simulink model "BMS_Model"  (R2023b)
settings: Solver=ode45  StartTime=0.0  StopTime=1180  RelTol=1e-3
values from neighbouring files (symbols this model uses):
  C1_LUT = [1913.6,12447,30609 ... (first row only)    [Cell_Data_Script.m]
  Capacity_LUT = [28.01,27.63,27.64]    [Cell_Data_Script.m]
  cell_area = cell_length*cell_width    (= 0.02678)    [Cell_Data_Script.m]
  cell_cp_heat = 830    [Cell_Data_Script.m]
  cell_mass = 0.354    [Cell_Data_Script.m]
  Em_LUT = [3.49,3.51,3.52;3.55,3.56,3.56 ... (first row only)    [Cell_Data_Script.m]
  h_conv = 10    [Cell_Data_Script.m]
  R0_LUT = [0.0117,0.0085,0.0090;0.0110,0.0085,0.0090 ... (first row only)    [Cell_Data_Script.m]
  R1_LUT = [0.0109,0.0029,0.0013;0.0069,0.0024,0.0012 ... (first row only)    [Cell_Data_Script.m]
  SOC_LUT = [0;0.1;0.25;0.5;0.75;0.9;1.0]    [Cell_Data_Script.m]
  T_init = 293.15    [Cell_Data_Script.m]
  Temperature_LUT = [278.15,293.15,313.15]    [Cell_Data_Script.m]
settings Model: Creator=marri  LastModifiedBy=marri

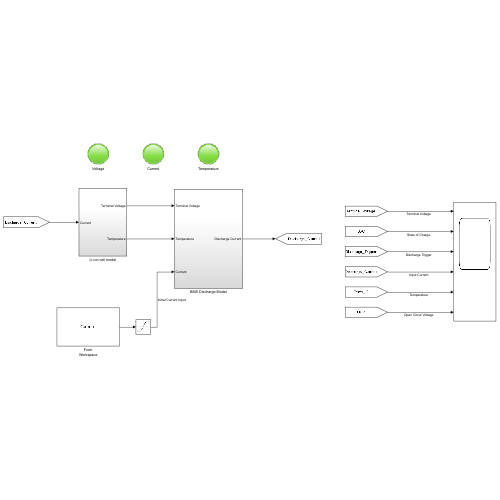
[thumbnail: Simulink's stored preview of the top-level diagram]
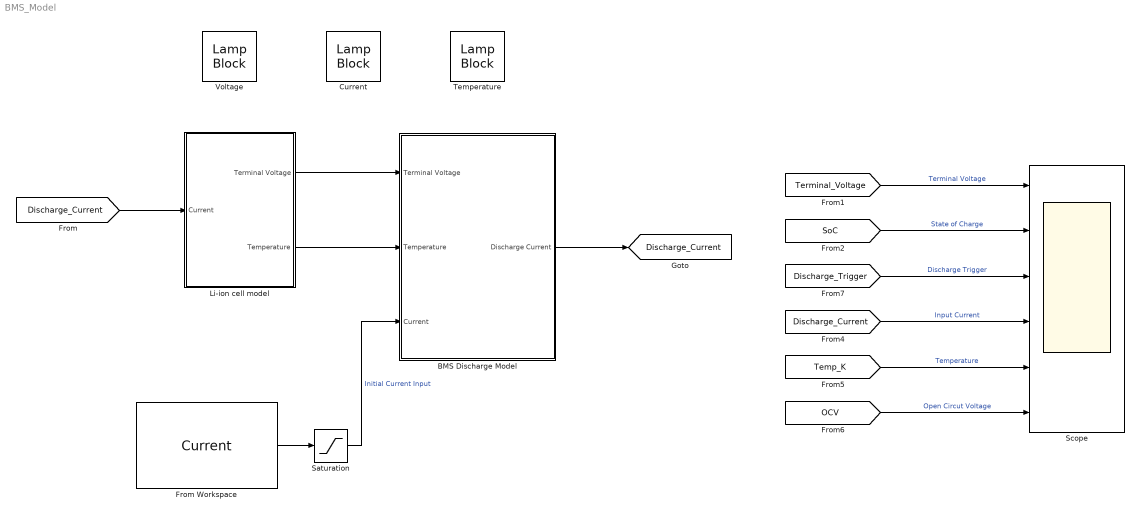
== system BMS_Model ==
  BMS Discharge Model : Subsystem
  Current : LampBlock  LabelPosition=Hide
  From Workspace : FromWorkspace  VariableName=Current
  Li-ion cell model : Subsystem
  Saturation : Saturate  UpperLimit=+inf  LowerLimit=0
  Scope : Scope  NumInputPorts=6
  Temperature : LampBlock  LabelPosition=Hide
  Voltage : LampBlock  LabelPosition=Hide
  tag scope: Discharge_Current=global
  wires:
  From Workspace/1 -> Saturation/1
  Saturation/1 -> BMS Discharge Model/3(Current)  "Initial Current Input"
  BMS Discharge Model/1(Discharge Current) -> [Discharge_Current]
  [Discharge_Current] -> Li-ion cell model/1(Current)
  Li-ion cell model/1(Terminal Voltage) -> BMS Discharge Model/1(Terminal Voltage)
  Li-ion cell model/2(Temperature) -> BMS Discharge Model/2(Temperature)
  [Terminal_Voltage] -> Scope/1  "Terminal Voltage"
  [SoC] -> Scope/2  "State of Charge"
  [Discharge_Current] -> Scope/4  "Input Current"
  [Temp_K] -> Scope/5  "Temperature"
  [OCV] -> Scope/6  "Open Circut Voltage"
  [Discharge_Trigger] -> Scope/3  "Discharge Trigger"

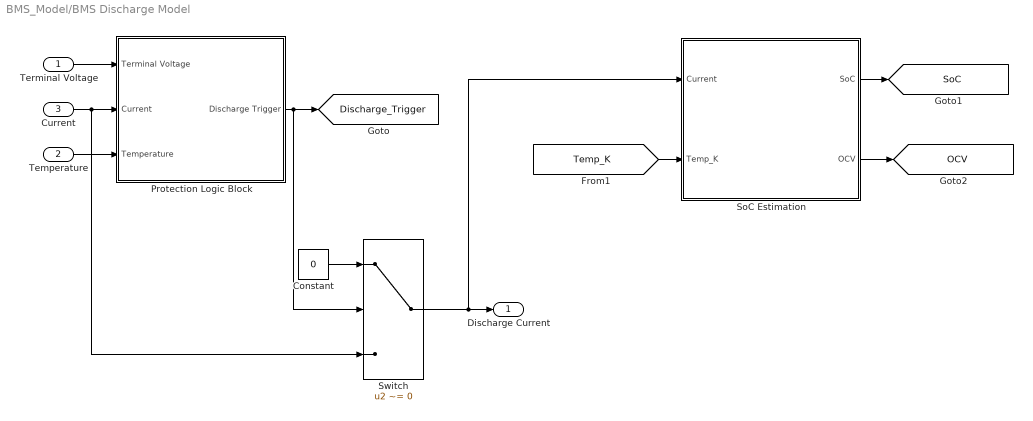
== system BMS_Model/BMS Discharge Model ==
  Terminal Voltage : Inport
  Temperature : Inport  Port=2
  Current : Inport  Port=3
  Constant : Constant  Value=0
  Protection Logic Block : Subsystem
  SoC Estimation : Subsystem
  Switch : Switch  Criteria=u2 ~= 0  SaturateOnIntegerOverflow=off  InputSameDT=off
  Discharge Current : Outport
  tag scope: Discharge_Trigger=global, OCV=global, SoC=global
  wires:
  Terminal Voltage/1 -> Protection Logic Block/1(Terminal Voltage)
  Current/1 -> Switch/3, Protection Logic Block/2(Current)
  Temperature/1 -> Protection Logic Block/3(Temperature)
  Protection Logic Block/1(Discharge Trigger) -> Switch/2, [Discharge_Trigger]
  Constant/1 -> Switch/1
  Switch/1 -> Discharge Current/1, SoC Estimation/1(Current)
  [Temp_K] -> SoC Estimation/2(Temp_K)
  SoC Estimation/1(SoC) -> [SoC]
  SoC Estimation/2(OCV) -> [OCV]

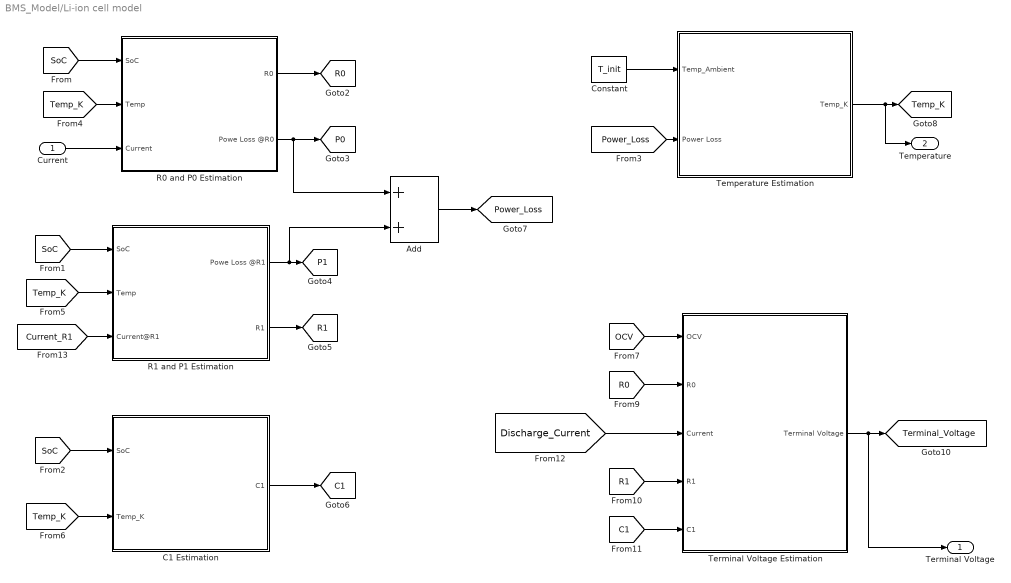
== system BMS_Model/Li-ion cell model ==
  Current : Inport
  Add : Sum
  C1 Estimation : Subsystem
  Constant : Constant  Value=T_init
  R0 and P0 Estimation : Subsystem
  R1 and P1 Estimation : Subsystem
  Temperature Estimation : Subsystem
  Terminal Voltage Estimation : Subsystem
  Terminal Voltage : Outport
  Temperature : Outport  Port=2
  tag scope: C1=global, P0=global, P1=global, Power_Loss=global, R0=global, R1=global, Temp_K=global, Terminal_Voltage=global
  wires:
  [SoC] -> R0 and P0 Estimation/1(SoC)
  [SoC] -> R1 and P1 Estimation/1(SoC)
  R0 and P0 Estimation/1(R0) -> [R0]
  R0 and P0 Estimation/2(Powe Loss @R0) -> Add/1, [P0]
  R1 and P1 Estimation/1(Powe Loss @R1) -> Add/2, [P1]
  R1 and P1 Estimation/2(R1) -> [R1]
  [SoC] -> C1 Estimation/1(SoC)
  C1 Estimation/1(C1) -> [C1]
  Add/1 -> [Power_Loss]
  Constant/1 -> Temperature Estimation/1(Temp_Ambient)
  [Power_Loss] -> Temperature Estimation/2(Power Loss)
  Temperature Estimation/1(Temp_K) -> Temperature/1, [Temp_K]
  [Temp_K] -> R0 and P0 Estimation/2(Temp)
  [Temp_K] -> R1 and P1 Estimation/2(Temp)
  [Temp_K] -> C1 Estimation/2(Temp_K)
  [R0] -> Terminal Voltage Estimation/2(R0)
  [R1] -> Terminal Voltage Estimation/4(R1)
  [C1] -> Terminal Voltage Estimation/5(C1)
  [Discharge_Current] -> Terminal Voltage Estimation/3(Current)
  [Current_R1] -> R1 and P1 Estimation/3(Current@R1)
  Terminal Voltage Estimation/1(Terminal Voltage) -> Terminal Voltage/1, [Terminal_Voltage]
  Current/1 -> R0 and P0 Estimation/3(Current)
  [OCV] -> Terminal Voltage Estimation/1(OCV)

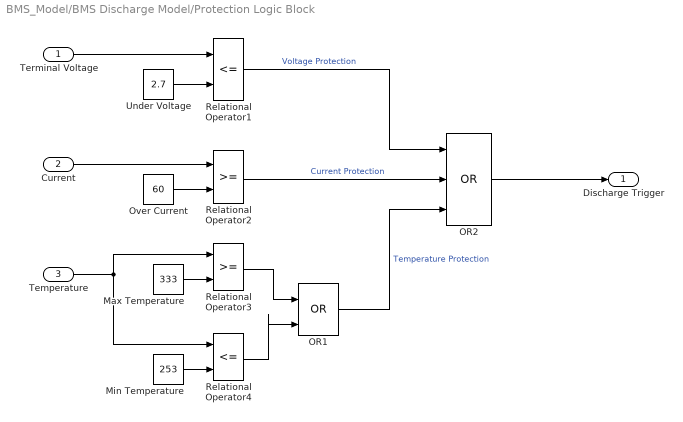
== system BMS_Model/BMS Discharge Model/Protection Logic Block ==
  Terminal Voltage : Inport
  Current : Inport  Port=2
  Temperature : Inport  Port=3
  Max Temperature : Constant  Value=333
  Min Temperature : Constant  Value=253
  OR1 : Logic  Operator=OR  IconShape=distinctive  AllPortsSameDT=off  OutDataTypeStr=boolean
  OR2 : Logic  Operator=OR  Inputs=3  IconShape=distinctive  AllPortsSameDT=off  OutDataTypeStr=boolean
  Over Current : Constant  Value=60
  Relational Operator1 : RelationalOperator  Operator=<=  OutDataTypeStr=boolean  RndMeth=Simplest  InputSameDT=off
  Relational Operator2 : RelationalOperator  OutDataTypeStr=boolean  RndMeth=Simplest  InputSameDT=off
  Relational Operator3 : RelationalOperator  OutDataTypeStr=boolean  RndMeth=Simplest  InputSameDT=off
  Relational Operator4 : RelationalOperator  Operator=<=  OutDataTypeStr=boolean  RndMeth=Simplest  InputSameDT=off
  Under Voltage : Constant  Value=2.7
  Discharge Trigger : Outport
  wires:
  Terminal Voltage/1 -> Relational Operator1/1
  Under Voltage/1 -> Relational Operator1/2
  Current/1 -> Relational Operator2/1
  Over Current/1 -> Relational Operator2/2
  Temperature/1 -> Relational Operator4/1, Relational Operator3/1
  Max Temperature/1 -> Relational Operator3/2
  Min Temperature/1 -> Relational Operator4/2
  Relational Operator3/1 -> OR1/1
  Relational Operator4/1 -> OR1/2
  Relational Operator2/1 -> OR2/2  "Current Protection"
  OR1/1 -> OR2/3  "Temperature Protection"
  OR2/1 -> Discharge Trigger/1
  Relational Operator1/1 -> OR2/1  "Voltage Protection"

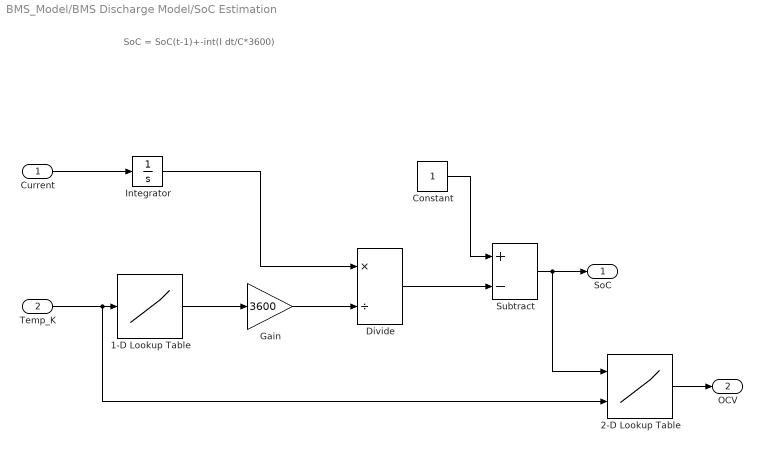
== system BMS_Model/BMS Discharge Model/SoC Estimation ==
  note: SoC = SoC(t-1)+-int(I dt/C*3600)
  Current : Inport
  Temp_K : Inport  Port=2
  1-D Lookup Table : Lookup_n-D  NumberOfTableDimensions=1  BreakpointsForDimension1=Temperature_LUT  Table=Capacity_LUT  InternalRulePriority=Speed  RndMeth=Simplest
  2-D Lookup Table : Lookup_n-D  BreakpointsForDimension1=SOC_LUT  BreakpointsForDimension2=Temperature_LUT  Table=Em_LUT  InternalRulePriority=Speed  RndMeth=Simplest
      settings: InputPortMap=u0,u1
  Constant : Constant
  Divide : Product  Inputs=*/
  Gain : Gain  Gain=3600
  Integrator : Integrator
  Subtract : Sum  Inputs=+-
  SoC : Outport
  OCV : Outport  Port=2
  wires:
  Temp_K/1 -> 2-D Lookup Table/2, 1-D Lookup Table/1
  1-D Lookup Table/1 -> Gain/1
  Current/1 -> Integrator/1
  Gain/1 -> Divide/2
  Integrator/1 -> Divide/1
  Divide/1 -> Subtract/2
  Constant/1 -> Subtract/1
  Subtract/1 -> 2-D Lookup Table/1, SoC/1
  2-D Lookup Table/1 -> OCV/1

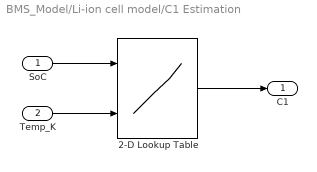
== system BMS_Model/Li-ion cell model/C1 Estimation ==
  SoC : Inport
  Temp_K : Inport  Port=2
  2-D Lookup Table : Lookup_n-D  BreakpointsForDimension1=SOC_LUT  BreakpointsForDimension2=Temperature_LUT  Table=C1_LUT  InternalRulePriority=Speed  RndMeth=Simplest
      settings: InputPortMap=u0,u1
  C1 : Outport
  wires:
  SoC/1 -> 2-D Lookup Table/1
  Temp_K/1 -> 2-D Lookup Table/2
  2-D Lookup Table/1 -> C1/1

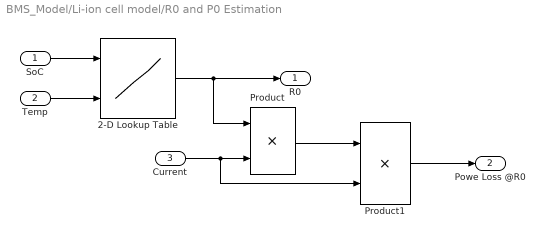
== system BMS_Model/Li-ion cell model/R0 and P0 Estimation ==
  SoC : Inport
  Temp : Inport  Port=2
  Current : Inport  Port=3
  2-D Lookup Table : Lookup_n-D  BreakpointsForDimension1=SOC_LUT  BreakpointsForDimension2=Temperature_LUT  Table=R0_LUT  InternalRulePriority=Speed  RndMeth=Simplest
      settings: InputPortMap=u0,u1
  Product : Product
  Product1 : Product
  R0 : Outport
  Powe Loss @R0 : Outport  Port=2
  wires:
  SoC/1 -> 2-D Lookup Table/1
  Temp/1 -> 2-D Lookup Table/2
  2-D Lookup Table/1 -> R0/1, Product/1
  Current/1 -> Product/2, Product1/2
  Product/1 -> Product1/1
  Product1/1 -> Powe Loss @R0/1

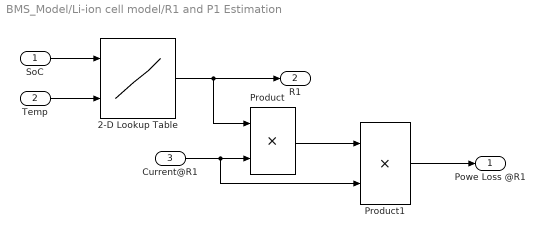
== system BMS_Model/Li-ion cell model/R1 and P1 Estimation ==
  SoC : Inport
  Temp : Inport  Port=2
  Current@R1 : Inport  Port=3
  2-D Lookup Table : Lookup_n-D  BreakpointsForDimension1=SOC_LUT  BreakpointsForDimension2=Temperature_LUT  Table=R1_LUT  InternalRulePriority=Speed  RndMeth=Simplest
      settings: InputPortMap=u0,u1
  Product : Product
  Product1 : Product
  Powe Loss @R1 : Outport
  R1 : Outport  Port=2
  wires:
  SoC/1 -> 2-D Lookup Table/1
  Temp/1 -> 2-D Lookup Table/2
  2-D Lookup Table/1 -> R1/1, Product/1
  Current@R1/1 -> Product/2, Product1/2
  Product/1 -> Product1/1
  Product1/1 -> Powe Loss @R1/1

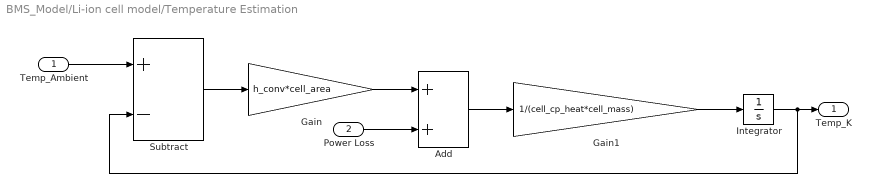
== system BMS_Model/Li-ion cell model/Temperature Estimation ==
  Temp_Ambient : Inport
  Power Loss : Inport  Port=2
  Add : Sum
  Gain : Gain  Gain=h_conv*cell_area
  Gain1 : Gain  Gain=1/(cell_cp_heat*cell_mass)
  Integrator : Integrator  InitialCondition=293.15
  Subtract : Sum  Inputs=+-
  Temp_K : Outport
  wires:
  Temp_Ambient/1 -> Subtract/1
  Subtract/1 -> Gain/1
  Gain/1 -> Add/1
  Power Loss/1 -> Add/2
  Add/1 -> Gain1/1
  Gain1/1 -> Integrator/1
  Integrator/1 -> Subtract/2, Temp_K/1

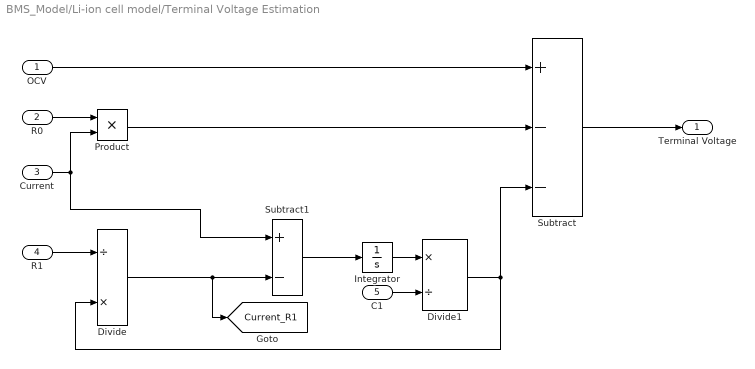
== system BMS_Model/Li-ion cell model/Terminal Voltage Estimation ==
  OCV : Inport
  R0 : Inport  Port=2
  Current : Inport  Port=3
  R1 : Inport  Port=4
  C1 : Inport  Port=5
  Divide : Product  Inputs=/*
  Divide1 : Product  Inputs=*/
  Integrator : Integrator
  Product : Product
  Subtract : Sum  Inputs=+--
  Subtract1 : Sum  Inputs=+-
  Terminal Voltage : Outport
  tag scope: Current_R1=global
  wires:
  OCV/1 -> Subtract/1
  R0/1 -> Product/1
  Current/1 -> Subtract1/1, Product/2
  Product/1 -> Subtract/2
  R1/1 -> Divide/1
  Divide/1 -> [Current_R1], Subtract1/2
  Subtract1/1 -> Integrator/1
  Integrator/1 -> Divide1/1
  C1/1 -> Divide1/2
  Divide1/1 -> Divide/2, Subtract/3
  Subtract/1 -> Terminal Voltage/1
